simulink model "CheckPosition"  (R2021a)
settings: Solver=VariableStepAuto  StartTime=0.0  StopTime=10.0  RelTol=1e-3
settings Model: Creator=kylec  LastModifiedBy=kylec

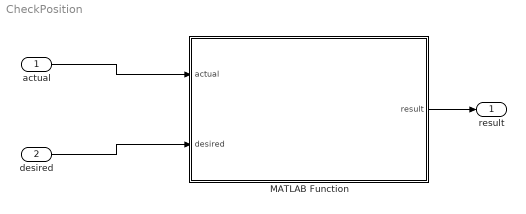
== system CheckPosition ==
  actual : Inport
  desired : Inport  Port=2
  MATLAB Function : MATLAB Function  TreatAsAtomicUnit=on
  result : Outport
  wires:
  actual/1 -> MATLAB Function/1(actual)
  desired/1 -> MATLAB Function/2(desired)
  MATLAB Function/1(result) -> result/1

== matlab function CheckPosition/MATLAB Function ==
  data: actual input; result output; desired input
function result = fcn(actual, desired)
    if abs(actual-desired)>0.0001
        result = 1;
    else
        result = 0; 
    end
 
end
